simulink model "expt2"  (R2021a)
settings: Solver=VariableStepAuto  StartTime=0.0  StopTime=50  RelTol=1e-3
settings Model: Creator=Kryptic  LastModifiedBy=Kryptic

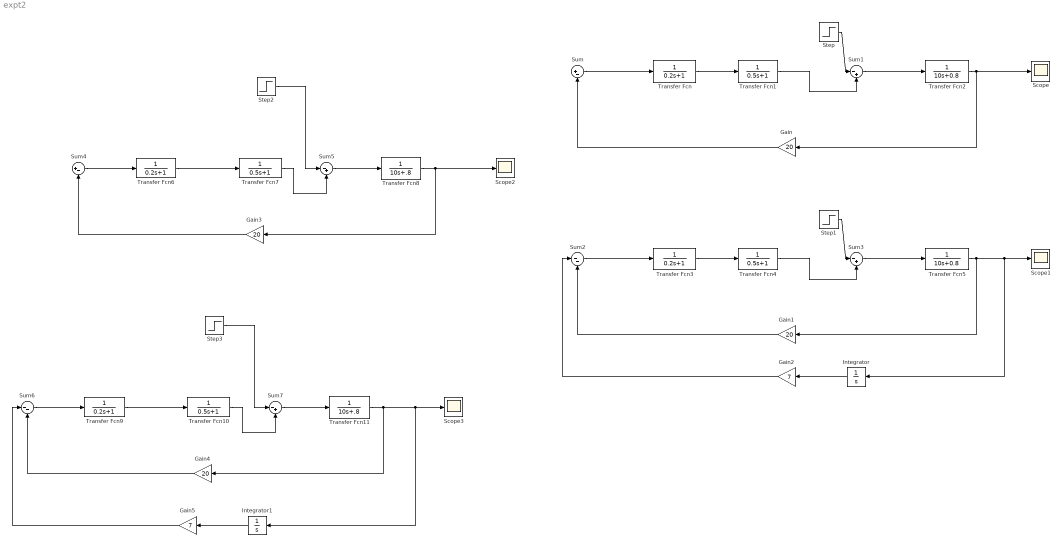
== system expt2 ==
  Gain{,1,3..4} (4 alike) : Gain  Gain=20
  Gain2 : Gain  Gain=7
  Gain5 : Gain  Gain=7
  Integrator : Integrator
  Integrator1 : Integrator
  Scope{,1..3} (4 alike) : Scope
  Step{,1..3} (4 alike) : Step  Time=0  After=0.2  SampleTime=0
  Sum : Sum  Inputs=|+-
  Sum{1,3,5,7} (4 alike) : Sum  Inputs=|-+
  Sum2 : Sum  Inputs=|--
  Sum4 : Sum  Inputs=|+-
  Sum6 : Sum  Inputs=|--
  Transfer Fcn{,3,6,9} (4 alike) : TransferFcn  Denominator=[0.2 1]
  Transfer Fcn{1,4,7,10} (4 alike) : TransferFcn  Denominator=[0.5 1]
  Transfer Fcn11 : TransferFcn  Denominator=[10 .8]
  Transfer Fcn2 : TransferFcn  Denominator=[10 0.8]
  Transfer Fcn5 : TransferFcn  Denominator=[10 0.8]
  Transfer Fcn8 : TransferFcn  Denominator=[10 .8]
  wires:
  Sum/1 -> Transfer Fcn/1
  Transfer Fcn/1 -> Transfer Fcn1/1
  Transfer Fcn1/1 -> Sum1/2
  Step/1 -> Sum1/1
  Sum1/1 -> Transfer Fcn2/1
  Transfer Fcn2/1 -> Scope/1, Gain/1
  Gain/1 -> Sum/2
  Gain1/1 -> Sum2/2
  Sum3/1 -> Transfer Fcn5/1
  Transfer Fcn4/1 -> Sum3/2
  Transfer Fcn3/1 -> Transfer Fcn4/1
  Sum2/1 -> Transfer Fcn3/1
  Step1/1 -> Sum3/1
  Transfer Fcn5/1 -> Integrator/1, Scope1/1, Gain1/1
  Integrator/1 -> Gain2/1
  Gain2/1 -> Sum2/1
  Sum4/1 -> Transfer Fcn6/1
  Transfer Fcn6/1 -> Transfer Fcn7/1
  Step2/1 -> Sum5/1
  Transfer Fcn7/1 -> Sum5/2
  Sum5/1 -> Transfer Fcn8/1
  Transfer Fcn8/1 -> Scope2/1, Gain3/1
  Gain3/1 -> Sum4/2
  Transfer Fcn9/1 -> Transfer Fcn10/1
  Transfer Fcn10/1 -> Sum7/2
  Step3/1 -> Sum7/1
  Transfer Fcn11/1 -> Integrator1/1, Scope3/1, Gain4/1
  Sum7/1 -> Transfer Fcn11/1
  Gain4/1 -> Sum6/2
  Sum6/1 -> Transfer Fcn9/1
  Integrator1/1 -> Gain5/1
  Gain5/1 -> Sum6/1
